simulink model "decoder8to256"  (R2020a)
settings: Solver=VariableStepAuto  StartTime=0.0  StopTime=10.0  RelTol=1e-3
(part 1 of 2)
settings Model: Creator=kishan  LastModifiedBy=kishan

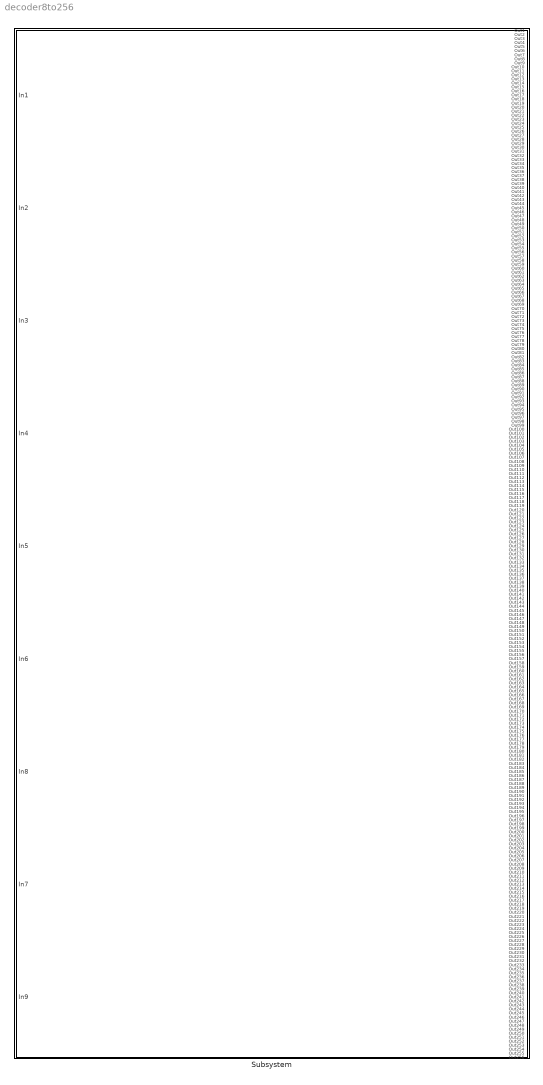
== system decoder8to256 ==
  Subsystem : Subsystem

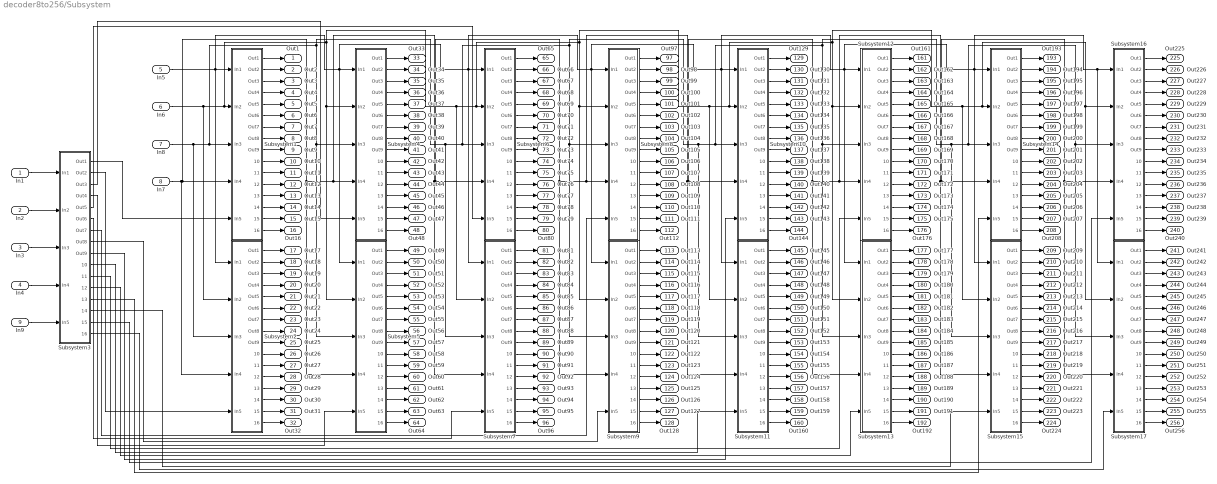
== system decoder8to256/Subsystem ==
  In1 : Inport
  In2 : Inport  Port=2
  In3 : Inport  Port=3
  In4 : Inport  Port=4
  In5 : Inport  Port=5
  In6 : Inport  Port=6
  In8 : Inport  Port=7
  In7 : Inport  Port=8
  In9 : Inport  Port=9
  Subsystem1 : Subsystem
  Subsystem10 : Subsystem
  Subsystem11 : Subsystem
  Subsystem12 : Subsystem
  Subsystem13 : Subsystem
  Subsystem14 : Subsystem
  Subsystem15 : Subsystem
  Subsystem16 : Subsystem
  Subsystem17 : Subsystem
  Subsystem2 : Subsystem
  Subsystem3 : Subsystem
  Subsystem4 : Subsystem
  Subsystem5 : Subsystem
  Subsystem6 : Subsystem
  Subsystem7 : Subsystem
  Subsystem8 : Subsystem
  Subsystem9 : Subsystem
  Out1 : Outport
  Out2 : Outport  Port=2
  Out3 : Outport  Port=3
  Out4 : Outport  Port=4
  Out5 : Outport  Port=5
  Out6 : Outport  Port=6
  Out7 : Outport  Port=7
  Out8 : Outport  Port=8
  Out9 : Outport  Port=9
  Out10 : Outport  Port=10
  Out11 : Outport  Port=11
  Out12 : Outport  Port=12
  Out13 : Outport  Port=13
  Out14 : Outport  Port=14
  Out15 : Outport  Port=15
  Out16 : Outport  Port=16
  Out17 : Outport  Port=17
  Out18 : Outport  Port=18
  Out19 : Outport  Port=19
  Out20 : Outport  Port=20
  Out21 : Outport  Port=21
  Out22 : Outport  Port=22
  Out23 : Outport  Port=23
  Out24 : Outport  Port=24
  Out25 : Outport  Port=25
  Out26 : Outport  Port=26
  Out27 : Outport  Port=27
  Out28 : Outport  Port=28
  Out29 : Outport  Port=29
  Out30 : Outport  Port=30
  Out31 : Outport  Port=31
  Out32 : Outport  Port=32
  Out33 : Outport  Port=33
  Out34 : Outport  Port=34
  Out35 : Outport  Port=35
  Out36 : Outport  Port=36
  Out37 : Outport  Port=37
  Out38 : Outport  Port=38
  Out39 : Outport  Port=39
  Out40 : Outport  Port=40
  Out41 : Outport  Port=41
  Out42 : Outport  Port=42
  Out43 : Outport  Port=43
  Out44 : Outport  Port=44
  Out45 : Outport  Port=45
  Out46 : Outport  Port=46
  Out47 : Outport  Port=47
  Out48 : Outport  Port=48
  Out49 : Outport  Port=49
  Out50 : Outport  Port=50
  Out51 : Outport  Port=51
  Out52 : Outport  Port=52
  Out53 : Outport  Port=53
  Out54 : Outport  Port=54
  Out55 : Outport  Port=55
  Out56 : Outport  Port=56
  Out57 : Outport  Port=57
  Out58 : Outport  Port=58
  Out59 : Outport  Port=59
  Out60 : Outport  Port=60
  Out61 : Outport  Port=61
  Out62 : Outport  Port=62
  Out63 : Outport  Port=63
  Out64 : Outport  Port=64
  Out65 : Outport  Port=65
  Out66 : Outport  Port=66
  Out67 : Outport  Port=67
  Out68 : Outport  Port=68
  Out69 : Outport  Port=69
  Out70 : Outport  Port=70
  Out71 : Outport  Port=71
  Out72 : Outport  Port=72
  Out73 : Outport  Port=73
  Out74 : Outport  Port=74
  Out75 : Outport  Port=75
  Out76 : Outport  Port=76
  Out77 : Outport  Port=77
  Out78 : Outport  Port=78
  Out79 : Outport  Port=79
  Out80 : Outport  Port=80
  Out81 : Outport  Port=81
  Out82 : Outport  Port=82
  Out83 : Outport  Port=83
  Out84 : Outport  Port=84
  Out85 : Outport  Port=85
  Out86 : Outport  Port=86
  Out87 : Outport  Port=87
  Out88 : Outport  Port=88
  Out89 : Outport  Port=89
  Out90 : Outport  Port=90
  Out91 : Outport  Port=91
  Out92 : Outport  Port=92
  Out93 : Outport  Port=93
  Out94 : Outport  Port=94
  Out95 : Outport  Port=95
  Out96 : Outport  Port=96
  Out97 : Outport  Port=97
  Out98 : Outport  Port=98
  Out99 : Outport  Port=99
  Out100 : Outport  Port=100
  Out101 : Outport  Port=101
  Out102 : Outport  Port=102
  Out103 : Outport  Port=103
  Out104 : Outport  Port=104
  Out105 : Outport  Port=105
  Out106 : Outport  Port=106
  Out107 : Outport  Port=107
  Out108 : Outport  Port=108
  Out109 : Outport  Port=109
  Out110 : Outport  Port=110
  Out111 : Outport  Port=111
  Out112 : Outport  Port=112
  Out113 : Outport  Port=113
  Out114 : Outport  Port=114
  Out115 : Outport  Port=115
  Out116 : Outport  Port=116
  Out117 : Outport  Port=117
  Out118 : Outport  Port=118
  Out119 : Outport  Port=119
  Out120 : Outport  Port=120
  Out121 : Outport  Port=121
  Out122 : Outport  Port=122
  Out123 : Outport  Port=123
  Out124 : Outport  Port=124
  Out125 : Outport  Port=125
  Out126 : Outport  Port=126
  Out127 : Outport  Port=127
  Out128 : Outport  Port=128
  Out129 : Outport  Port=129
  Out130 : Outport  Port=130
  Out131 : Outport  Port=131
  Out132 : Outport  Port=132
  Out133 : Outport  Port=133
  Out134 : Outport  Port=134
  Out135 : Outport  Port=135
  Out136 : Outport  Port=136
  Out137 : Outport  Port=137
  Out138 : Outport  Port=138
  Out139 : Outport  Port=139
  Out140 : Outport  Port=140
  Out141 : Outport  Port=141
  Out142 : Outport  Port=142
  Out143 : Outport  Port=143
  Out144 : Outport  Port=144
  Out145 : Outport  Port=145
  Out146 : Outport  Port=146
  Out147 : Outport  Port=147
  Out148 : Outport  Port=148
  Out149 : Outport  Port=149
  Out150 : Outport  Port=150
  Out151 : Outport  Port=151
  Out152 : Outport  Port=152
  Out153 : Outport  Port=153
  Out154 : Outport  Port=154
  Out155 : Outport  Port=155
  Out156 : Outport  Port=156
  Out157 : Outport  Port=157
  Out158 : Outport  Port=158
  Out159 : Outport  Port=159
  Out160 : Outport  Port=160
  Out161 : Outport  Port=161
  Out162 : Outport  Port=162
  Out163 : Outport  Port=163
  Out164 : Outport  Port=164
  Out165 : Outport  Port=165
  Out166 : Outport  Port=166
  Out167 : Outport  Port=167
  Out168 : Outport  Port=168
  Out169 : Outport  Port=169
  Out170 : Outport  Port=170
  Out171 : Outport  Port=171
  Out172 : Outport  Port=172
  Out173 : Outport  Port=173
  Out174 : Outport  Port=174
  Out175 : Outport  Port=175
  Out176 : Outport  Port=176
  Out177 : Outport  Port=177
  Out178 : Outport  Port=178
  Out179 : Outport  Port=179
  Out180 : Outport  Port=180
  Out181 : Outport  Port=181
  Out182 : Outport  Port=182
  Out183 : Outport  Port=183
  Out184 : Outport  Port=184
  Out185 : Outport  Port=185
  Out186 : Outport  Port=186
  Out187 : Outport  Port=187
  Out188 : Outport  Port=188
  Out189 : Outport  Port=189
  Out190 : Outport  Port=190
  Out191 : Outport  Port=191
  Out192 : Outport  Port=192
  Out193 : Outport  Port=193
  Out194 : Outport  Port=194
  Out195 : Outport  Port=195
  Out196 : Outport  Port=196
  Out197 : Outport  Port=197
  Out198 : Outport  Port=198
  Out199 : Outport  Port=199
  Out200 : Outport  Port=200
  Out201 : Outport  Port=201
  Out202 : Outport  Port=202
  Out203 : Outport  Port=203
  Out204 : Outport  Port=204
  Out205 : Outport  Port=205
  Out206 : Outport  Port=206
  Out207 : Outport  Port=207
  Out208 : Outport  Port=208
  Out209 : Outport  Port=209
  Out210 : Outport  Port=210
  Out211 : Outport  Port=211
  Out212 : Outport  Port=212
  Out213 : Outport  Port=213
  Out214 : Outport  Port=214
  Out215 : Outport  Port=215
  Out216 : Outport  Port=216
  Out217 : Outport  Port=217
  Out218 : Outport  Port=218
  Out219 : Outport  Port=219
  Out220 : Outport  Port=220
  Out221 : Outport  Port=221
  Out222 : Outport  Port=222
  Out223 : Outport  Port=223
  Out224 : Outport  Port=224
  Out225 : Outport  Port=225
  Out226 : Outport  Port=226
  Out227 : Outport  Port=227
  Out228 : Outport  Port=228
  Out229 : Outport  Port=229
  Out230 : Outport  Port=230
  Out231 : Outport  Port=231
  Out232 : Outport  Port=232
  Out233 : Outport  Port=233
  Out234 : Outport  Port=234
  Out235 : Outport  Port=235
  Out236 : Outport  Port=236
  Out237 : Outport  Port=237
  Out238 : Outport  Port=238
  Out239 : Outport  Port=239
  Out240 : Outport  Port=240
  Out241 : Outport  Port=241
  Out242 : Outport  Port=242
  Out243 : Outport  Port=243
  Out244 : Outport  Port=244
  Out245 : Outport  Port=245
  Out246 : Outport  Port=246
  Out247 : Outport  Port=247
  Out248 : Outport  Port=248
  Out249 : Outport  Port=249
  Out250 : Outport  Port=250
  Out251 : Outport  Port=251
  Out252 : Outport  Port=252
  Out253 : Outport  Port=253
  Out254 : Outport  Port=254
  Out255 : Outport  Port=255
  Out256 : Outport  Port=256
  wires:
  Subsystem17/5(Out5) -> Out245/1
  Subsystem15/13(Out13) -> Out221/1
  Subsystem5/12(Out12) -> Out60/1
  Subsystem6/8(Out8) -> Out72/1
  Subsystem10/7(Out7) -> Out135/1
  Subsystem13/13(Out13) -> Out189/1
  Subsystem14/10(Out10) -> Out202/1
  Subsystem11/5(Out5) -> Out149/1
  Subsystem10/5(Out5) -> Out133/1
  Subsystem7/14(Out14) -> Out94/1
  Subsystem7/2(Out2) -> Out82/1
  Subsystem12/7(Out7) -> Out167/1
  Subsystem7/10(Out10) -> Out90/1
  Subsystem8/12(Out12) -> Out108/1
  Subsystem12/1(Out1) -> Out161/1
  Subsystem17/4(Out4) -> Out244/1
  Subsystem7/15(Out15) -> Out95/1
  Subsystem10/13(Out13) -> Out141/1
  Subsystem3/12(Out12) -> Subsystem13/5(In5)
  Subsystem5/14(Out14) -> Out62/1
  Subsystem15/15(Out15) -> Out223/1
  Subsystem6/11(Out11) -> Out75/1
  Subsystem14/16(Out16) -> Out208/1
  Subsystem6/2(Out2) -> Out66/1
  Subsystem7/16(Out16) -> Out96/1
  Subsystem13/12(Out12) -> Out188/1
  Subsystem8/9(Out9) -> Out105/1
  Subsystem11/16(Out16) -> Out160/1
  Subsystem4/7(Out7) -> Out39/1
  Subsystem6/3(Out3) -> Out67/1
  In2/1 -> Subsystem3/2(In2)
  In4/1 -> Subsystem3/4(In4)
  Subsystem1/4(Out4) -> Out4/1
  Subsystem8/1(Out1) -> Out97/1
  Subsystem6/9(Out9) -> Out73/1
  Subsystem11/15(Out15) -> Out159/1
  Subsystem11/6(Out6) -> Out150/1
  Subsystem3/9(Out9) -> Subsystem10/5(In5)
  Subsystem17/10(Out10) -> Out250/1
  Subsystem9/4(Out4) -> Out116/1
  Subsystem9/8(Out8) -> Out120/1
  Subsystem11/7(Out7) -> Out151/1
  Subsystem9/6(Out6) -> Out118/1
  Subsystem4/4(Out4) -> Out36/1
  Subsystem16/1(Out1) -> Out225/1
  Subsystem9/14(Out14) -> Out126/1
  Subsystem7/4(Out4) -> Out84/1
  Subsystem9/16(Out16) -> Out128/1
  Subsystem1/14(Out14) -> Out14/1
  Subsystem12/14(Out14) -> Out174/1
  Subsystem6/12(Out12) -> Out76/1
  Subsystem16/11(Out11) -> Out235/1
  Subsystem15/12(Out12) -> Out220/1
  Subsystem8/7(Out7) -> Out103/1
  Subsystem13/6(Out6) -> Out182/1
  Subsystem5/4(Out4) -> Out52/1
  Subsystem14/8(Out8) -> Out200/1
  Subsystem14/1(Out1) -> Out193/1
  Subsystem11/3(Out3) -> Out147/1
  Subsystem16/16(Out16) -> Out240/1
  Subsystem4/6(Out6) -> Out38/1
  Subsystem5/6(Out6) -> Out54/1
  Subsystem15/16(Out16) -> Out224/1
  Subsystem2/14(Out14) -> Out30/1
  Subsystem3/7(Out7) -> Subsystem8/5(In5)
  Subsystem3/2(Out2) -> Subsystem2/5(In5)
  Subsystem13/2(Out2) -> Out178/1
  Subsystem7/7(Out7) -> Out87/1
  Subsystem1/3(Out3) -> Out3/1
  Subsystem4/3(Out3) -> Out35/1
  Subsystem11/2(Out2) -> Out146/1
  In5/1 -> Subsystem17/1(In1), Subsystem16/1(In1), Subsystem15/1(In1), Subsystem14/1(In1), Subsystem13/1(In1), Subsystem12/1(In1), Subsystem11/1(In1), Subsystem10/1(In1), Subsystem9/1(In1), Subsystem8/1(In1), Subsystem7/1(In1), Subsystem6/1(In1), Subsystem5/1(In1), Subsystem4/1(In1), Subsystem2/1(In1), Subsystem1/1(In1)
  Subsystem17/15(Out15) -> Out255/1
  Subsystem8/13(Out13) -> Out109/1
  Subsystem3/14(Out14) -> Subsystem15/5(In5)
  Subsystem3/10(Out10) -> Subsystem11/5(In5)
  Subsystem13/5(Out5) -> Out181/1
  Subsystem14/11(Out11) -> Out203/1
  Subsystem6/4(Out4) -> Out68/1
  Subsystem10/6(Out6) -> Out134/1
  Subsystem2/3(Out3) -> Out19/1
  Subsystem12/9(Out9) -> Out169/1
  Subsystem2/9(Out9) -> Out25/1
  Subsystem13/16(Out16) -> Out192/1
  Subsystem3/8(Out8) -> Subsystem9/5(In5)
  Subsystem15/8(Out8) -> Out216/1
  Subsystem14/4(Out4) -> Out196/1
  Subsystem5/8(Out8) -> Out56/1
  Subsystem9/12(Out12) -> Out124/1
  Subsystem16/7(Out7) -> Out231/1
  Subsystem9/1(Out1) -> Out113/1
  Subsystem16/3(Out3) -> Out227/1
  Subsystem13/15(Out15) -> Out191/1
  Subsystem17/2(Out2) -> Out242/1
  Subsystem1/6(Out6) -> Out6/1
  Subsystem2/4(Out4) -> Out20/1
  Subsystem16/8(Out8) -> Out232/1
  In3/1 -> Subsystem3/3(In3)
  Subsystem1/8(Out8) -> Out8/1
  Subsystem4/9(Out9) -> Out41/1
  Subsystem5/5(Out5) -> Out53/1
  Subsystem17/8(Out8) -> Out248/1
  Subsystem7/1(Out1) -> Out81/1
  Subsystem14/6(Out6) -> Out198/1
  Subsystem2/10(Out10) -> Out26/1
  Subsystem15/1(Out1) -> Out209/1
  Subsystem17/3(Out3) -> Out243/1
  Subsystem9/3(Out3) -> Out115/1
  Subsystem3/6(Out6) -> Subsystem7/5(In5)
  Subsystem7/13(Out13) -> Out93/1
  Subsystem17/12(Out12) -> Out252/1
  Subsystem9/2(Out2) -> Out114/1
  Subsystem6/16(Out16) -> Out80/1
  Subsystem11/13(Out13) -> Out157/1
  Subsystem10/1(Out1) -> Out129/1
  Subsystem7/9(Out9) -> Out89/1
  Subsystem15/6(Out6) -> Out214/1
  Subsystem17/11(Out11) -> Out251/1
  Subsystem12/16(Out16) -> Out176/1
  Subsystem4/12(Out12) -> Out44/1
  Subsystem2/5(Out5) -> Out21/1
  Subsystem8/16(Out16) -> Out112/1
  Subsystem16/4(Out4) -> Out228/1
  Subsystem6/10(Out10) -> Out74/1
  Subsystem5/16(Out16) -> Out64/1
  Subsystem5/11(Out11) -> Out59/1
  Subsystem1/12(Out12) -> Out12/1
  Subsystem11/12(Out12) -> Out156/1
  Subsystem1/7(Out7) -> Out7/1
  Subsystem14/13(Out13) -> Out205/1
  Subsystem2/15(Out15) -> Out31/1
  Subsystem10/10(Out10) -> Out138/1
  Subsystem13/4(Out4) -> Out180/1
  Subsystem11/10(Out10) -> Out154/1
  Subsystem11/1(Out1) -> Out145/1
  Subsystem3/16(Out16) -> Subsystem17/5(In5)
  Subsystem7/6(Out6) -> Out86/1
  Subsystem13/7(Out7) -> Out183/1
  Subsystem6/5(Out5) -> Out69/1
  Subsystem16/6(Out6) -> Out230/1
  Subsystem10/15(Out15) -> Out143/1
  Subsystem17/1(Out1) -> Out241/1
  Subsystem9/5(Out5) -> Out117/1
  Subsystem16/5(Out5) -> Out229/1
  Subsystem16/9(Out9) -> Out233/1
  Subsystem14/9(Out9) -> Out201/1
  Subsystem4/8(Out8) -> Out40/1
  Subsystem1/5(Out5) -> Out5/1
  Subsystem14/12(Out12) -> Out204/1
  Subsystem9/7(Out7) -> Out119/1
  Subsystem17/14(Out14) -> Out254/1
  Subsystem14/15(Out15) -> Out207/1
  Subsystem15/10(Out10) -> Out218/1
  Subsystem9/13(Out13) -> Out125/1
  Subsystem2/6(Out6) -> Out22/1
  Subsystem11/9(Out9) -> Out153/1
  Subsystem16/2(Out2) -> Out226/1
  Subsystem12/2(Out2) -> Out162/1
  Subsystem15/11(Out11) -> Out219/1
  Subsystem14/5(Out5) -> Out197/1
  Subsystem13/11(Out11) -> Out187/1
  In9/1 -> Subsystem3/5(In5)
  Subsystem16/12(Out12) -> Out236/1
  Subsystem1/1(Out1) -> Out1/1
  Subsystem12/13(Out13) -> Out173/1
  Subsystem9/9(Out9) -> Out121/1
  Subsystem17/9(Out9) -> Out249/1
  Subsystem12/10(Out10) -> Out170/1
  Subsystem15/3(Out3) -> Out211/1
  Subsystem3/13(Out13) -> Subsystem14/5(In5)
  Subsystem4/14(Out14) -> Out46/1
  In7/1 -> Subsystem17/4(In4), Subsystem16/4(In4), Subsystem14/4(In4), Subsystem15/4(In4), Subsystem12/4(In4), Subsystem13/4(In4), Subsystem10/4(In4), Subsystem11/4(In4), Subsystem8/4(In4), Subsystem9/4(In4), Subsystem6/4(In4), Subsystem7/4(In4), Subsystem4/4(In4), Subsystem5/4(In4), Subsystem1/4(In4), Subsystem2/4(In4)
  Subsystem15/9(Out9) -> Out217/1
  Subsystem10/3(Out3) -> Out131/1
  Subsystem1/11(Out11) -> Out11/1
  Subsystem6/14(Out14) -> Out78/1
  Subsystem5/2(Out2) -> Out50/1
  Subsystem10/16(Out16) -> Out144/1
  Subsystem5/9(Out9) -> Out57/1
  Subsystem1/10(Out10) -> Out10/1
  Subsystem14/7(Out7) -> Out199/1
  Subsystem8/5(Out5) -> Out101/1
  Subsystem16/10(Out10) -> Out234/1
  Subsystem15/4(Out4) -> Out212/1
  Subsystem17/6(Out6) -> Out246/1
  Subsystem12/11(Out11) -> Out171/1
  Subsystem12/6(Out6) -> Out166/1
  Subsystem9/11(Out11) -> Out123/1
  Subsystem1/13(Out13) -> Out13/1
  Subsystem5/3(Out3) -> Out51/1
  Subsystem8/14(Out14) -> Out110/1
  Subsystem4/5(Out5) -> Out37/1
  Subsystem17/16(Out16) -> Out256/1
  Subsystem10/9(Out9) -> Out137/1
  Subsystem17/7(Out7) -> Out247/1
  Subsystem13/8(Out8) -> Out184/1
  Subsystem4/2(Out2) -> Out34/1
  Subsystem3/4(Out4) -> Subsystem5/5(In5)
  Subsystem11/4(Out4) -> Out148/1
  Subsystem10/14(Out14) -> Out142/1
  Subsystem4/11(Out11) -> Out43/1
  Subsystem8/15(Out15) -> Out111/1
  Subsystem2/7(Out7) -> Out23/1
  Subsystem9/15(Out15) -> Out127/1
  Subsystem3/1(Out1) -> Subsystem1/5(In5)
  Subsystem5/13(Out13) -> Out61/1
  Subsystem6/13(Out13) -> Out77/1
  Subsystem16/14(Out14) -> Out238/1
  Subsystem13/10(Out10) -> Out186/1
  In8/1 -> Subsystem1/3(In3), Subsystem5/3(In3), Subsystem4/3(In3), Subsystem6/3(In3), Subsystem9/3(In3), Subsystem8/3(In3), Subsystem10/3(In3), Subsystem13/3(In3), Subsystem12/3(In3), Subsystem14/3(In3), Subsystem17/3(In3), Subsystem16/3(In3), Subsystem15/3(In3), Subsystem11/3(In3), Subsystem7/3(In3), Subsystem2/3(In3)
  Subsystem1/15(Out15) -> Out15/1
  Subsystem12/15(Out15) -> Out175/1
  Subsystem8/10(Out10) -> Out106/1
  Subsystem7/8(Out8) -> Out88/1
  Subsystem2/1(Out1) -> Out17/1
  Subsystem10/2(Out2) -> Out130/1
  Subsystem11/11(Out11) -> Out155/1
  Subsystem12/5(Out5) -> Out165/1
  Subsystem9/10(Out10) -> Out122/1
  Subsystem1/2(Out2) -> Out2/1
  Subsystem6/6(Out6) -> Out70/1
  Subsystem4/16(Out16) -> Out48/1
  Subsystem2/8(Out8) -> Out24/1
  Subsystem2/12(Out12) -> Out28/1
  Subsystem6/15(Out15) -> Out79/1
  Subsystem8/3(Out3) -> Out99/1
  Subsystem17/13(Out13) -> Out253/1
  Subsystem15/14(Out14) -> Out222/1
  Subsystem7/5(Out5) -> Out85/1
  Subsystem8/2(Out2) -> Out98/1
  Subsystem14/2(Out2) -> Out194/1
  Subsystem13/1(Out1) -> Out177/1
  Subsystem15/5(Out5) -> Out213/1
  Subsystem11/14(Out14) -> Out158/1
  Subsystem10/8(Out8) -> Out136/1
  Subsystem13/14(Out14) -> Out190/1
  In6/1 -> Subsystem5/2(In2), Subsystem4/2(In2), Subsystem9/2(In2), Subsystem8/2(In2), Subsystem13/2(In2), Subsystem12/2(In2), Subsystem17/2(In2), Subsystem16/2(In2), Subsystem14/2(In2), Subsystem15/2(In2), Subsystem10/2(In2), Subsystem11/2(In2), Subsystem6/2(In2), Subsystem7/2(In2), Subsystem1/2(In2), Subsystem2/2(In2)
  Subsystem11/8(Out8) -> Out152/1
  Subsystem8/6(Out6) -> Out102/1
  Subsystem8/4(Out4) -> Out100/1
  Subsystem15/7(Out7) -> Out215/1
  Subsystem4/15(Out15) -> Out47/1
  Subsystem12/12(Out12) -> Out172/1
  Subsystem15/2(Out2) -> Out210/1
  Subsystem16/13(Out13) -> Out237/1
  Subsystem6/1(Out1) -> Out65/1
  Subsystem16/15(Out15) -> Out239/1
  Subsystem12/3(Out3) -> Out163/1
  Subsystem5/10(Out10) -> Out58/1
  In1/1 -> Subsystem3/1(In1)
  Subsystem13/3(Out3) -> Out179/1
  Subsystem5/7(Out7) -> Out55/1
  Subsystem3/3(Out3) -> Subsystem4/5(In5)
  Subsystem4/13(Out13) -> Out45/1
  Subsystem2/2(Out2) -> Out18/1
  Subsystem2/16(Out16) -> Out32/1
  Subsystem4/10(Out10) -> Out42/1
  Subsystem7/12(Out12) -> Out92/1
  Subsystem1/16(Out16) -> Out16/1
  Subsystem2/11(Out11) -> Out27/1
  Subsystem10/11(Out11) -> Out139/1
  Subsystem12/4(Out4) -> Out164/1
  Subsystem14/3(Out3) -> Out195/1
  Subsystem5/1(Out1) -> Out49/1
  Subsystem8/11(Out11) -> Out107/1
  Subsystem10/12(Out12) -> Out140/1
  Subsystem2/13(Out13) -> Out29/1
  Subsystem12/8(Out8) -> Out168/1
  Subsystem1/9(Out9) -> Out9/1
  Subsystem10/4(Out4) -> Out132/1
  Subsystem13/9(Out9) -> Out185/1
  Subsystem3/15(Out15) -> Subsystem16/5(In5)
  Subsystem7/3(Out3) -> Out83/1
  Subsystem6/7(Out7) -> Out71/1
  Subsystem7/11(Out11) -> Out91/1
  Subsystem5/15(Out15) -> Out63/1
  Subsystem3/11(Out11) -> Subsystem12/5(In5)
  Subsystem14/14(Out14) -> Out206/1
  Subsystem4/1(Out1) -> Out33/1
  Subsystem3/5(Out5) -> Subsystem6/5(In5)
  Subsystem8/8(Out8) -> Out104/1

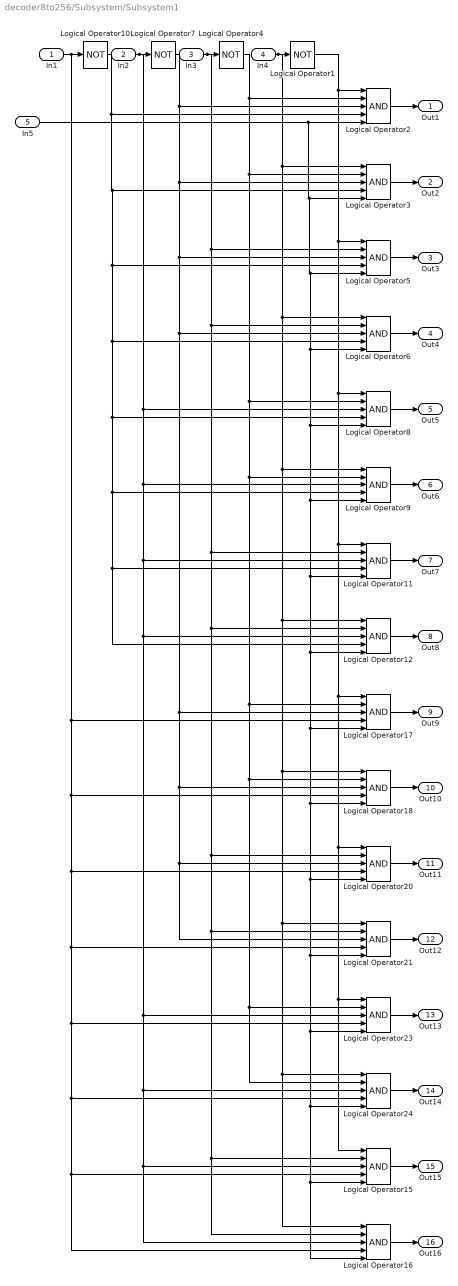
== system decoder8to256/Subsystem/Subsystem1 ==
  In1 : Inport
  In2 : Inport  Port=2
  In3 : Inport  Port=3
  In4 : Inport  Port=4
  In5 : Inport  Port=5
  Logical Operator{1,4,7,10} (4 alike) : Logic  Operator=NOT  AllPortsSameDT=off  OutDataTypeStr=boolean
  Logical Operator{2..3,5..6,8..9,11..12,15..18,20..21,23..24} (16 alike) : Logic  Inputs=5  AllPortsSameDT=off  OutDataTypeStr=boolean
  Out1 : Outport
  Out2 : Outport  Port=2
  Out3 : Outport  Port=3
  Out4 : Outport  Port=4
  Out5 : Outport  Port=5
  Out6 : Outport  Port=6
  Out7 : Outport  Port=7
  Out8 : Outport  Port=8
  Out9 : Outport  Port=9
  Out10 : Outport  Port=10
  Out11 : Outport  Port=11
  Out12 : Outport  Port=12
  Out13 : Outport  Port=13
  Out14 : Outport  Port=14
  Out15 : Outport  Port=15
  Out16 : Outport  Port=16
  wires:
  Logical Operator11/1 -> Out7/1
  Logical Operator12/1 -> Out8/1
  Logical Operator18/1 -> Out10/1
  In2/1 -> Logical Operator16/3, Logical Operator15/3, Logical Operator24/3, Logical Operator23/3, Logical Operator12/3, Logical Operator11/3, Logical Operator9/3, Logical Operator8/3, Logical Operator7/1
  In3/1 -> Logical Operator11/2, Logical Operator15/2, Logical Operator16/2, Logical Operator21/2, Logical Operator20/2, Logical Operator12/2, Logical Operator6/2, Logical Operator5/2, Logical Operator4/1
  Logical Operator24/1 -> Out14/1
  In4/1 -> Logical Operator16/1, Logical Operator24/1, Logical Operator21/1, Logical Operator18/1, Logical Operator12/1, Logical Operator9/1, Logical Operator6/1, Logical Operator3/1, Logical Operator1/1
  Logical Operator10/1 -> Logical Operator12/4, Logical Operator11/4, Logical Operator9/4, Logical Operator8/4, Logical Operator6/4, Logical Operator5/4, Logical Operator3/4, Logical Operator2/4
  Logical Operator9/1 -> Out6/1
  In5/1 -> Logical Operator16/5, Logical Operator15/5, Logical Operator24/5, Logical Operator23/5, Logical Operator21/5, Logical Operator20/5, Logical Operator18/5, Logical Operator17/5, Logical Operator12/5, Logical Operator11/5, Logical Operator9/5, Logical Operator8/5, Logical Operator6/5, Logical Operator5/5, Logical Operator3/5, Logical Operator2/5
  Logical Operator5/1 -> Out3/1
  Logical Operator1/1 -> Logical Operator15/1, Logical Operator23/1, Logical Operator20/1, Logical Operator17/1, Logical Operator11/1, Logical Operator8/1, Logical Operator5/1, Logical Operator2/1
  Logical Operator2/1 -> Out1/1
  Logical Operator21/1 -> Out12/1
  Logical Operator8/1 -> Out5/1
  Logical Operator7/1 -> Logical Operator21/3, Logical Operator20/3, Logical Operator18/3, Logical Operator17/3, Logical Operator6/3, Logical Operator5/3, Logical Operator3/3, Logical Operator2/3
  Logical Operator16/1 -> Out16/1
  Logical Operator15/1 -> Out15/1
  In1/1 -> Logical Operator17/4, Logical Operator18/4, Logical Operator20/4, Logical Operator21/4, Logical Operator23/4, Logical Operator24/4, Logical Operator15/4, Logical Operator16/4, Logical Operator10/1
  Logical Operator3/1 -> Out2/1
  Logical Operator20/1 -> Out11/1
  Logical Operator6/1 -> Out4/1
  Logical Operator23/1 -> Out13/1
  Logical Operator4/1 -> Logical Operator24/2, Logical Operator23/2, Logical Operator18/2, Logical Operator17/2, Logical Operator9/2, Logical Operator8/2, Logical Operator3/2, Logical Operator2/2
  Logical Operator17/1 -> Out9/1

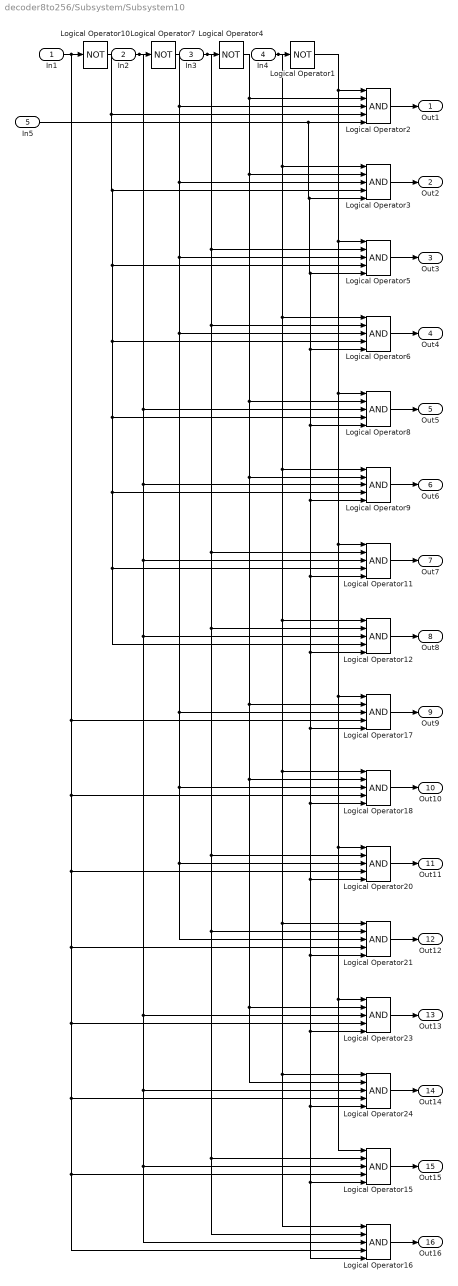
== system decoder8to256/Subsystem/Subsystem10 ==
  In1 : Inport
  In2 : Inport  Port=2
  In3 : Inport  Port=3
  In4 : Inport  Port=4
  In5 : Inport  Port=5
  Logical Operator{1,4,7,10} (4 alike) : Logic  Operator=NOT  AllPortsSameDT=off  OutDataTypeStr=boolean
  Logical Operator{2..3,5..6,8..9,11..12,15..18,20..21,23..24} (16 alike) : Logic  Inputs=5  AllPortsSameDT=off  OutDataTypeStr=boolean
  Out1 : Outport
  Out2 : Outport  Port=2
  Out3 : Outport  Port=3
  Out4 : Outport  Port=4
  Out5 : Outport  Port=5
  Out6 : Outport  Port=6
  Out7 : Outport  Port=7
  Out8 : Outport  Port=8
  Out9 : Outport  Port=9
  Out10 : Outport  Port=10
  Out11 : Outport  Port=11
  Out12 : Outport  Port=12
  Out13 : Outport  Port=13
  Out14 : Outport  Port=14
  Out15 : Outport  Port=15
  Out16 : Outport  Port=16
  wires:
  Logical Operator11/1 -> Out7/1
  Logical Operator12/1 -> Out8/1
  Logical Operator18/1 -> Out10/1
  In2/1 -> Logical Operator16/3, Logical Operator15/3, Logical Operator24/3, Logical Operator23/3, Logical Operator12/3, Logical Operator11/3, Logical Operator9/3, Logical Operator8/3, Logical Operator7/1
  In3/1 -> Logical Operator11/2, Logical Operator15/2, Logical Operator16/2, Logical Operator21/2, Logical Operator20/2, Logical Operator12/2, Logical Operator6/2, Logical Operator5/2, Logical Operator4/1
  Logical Operator24/1 -> Out14/1
  In4/1 -> Logical Operator16/1, Logical Operator24/1, Logical Operator21/1, Logical Operator18/1, Logical Operator12/1, Logical Operator9/1, Logical Operator6/1, Logical Operator3/1, Logical Operator1/1
  Logical Operator10/1 -> Logical Operator12/4, Logical Operator11/4, Logical Operator9/4, Logical Operator8/4, Logical Operator6/4, Logical Operator5/4, Logical Operator3/4, Logical Operator2/4
  Logical Operator9/1 -> Out6/1
  In5/1 -> Logical Operator16/5, Logical Operator15/5, Logical Operator24/5, Logical Operator23/5, Logical Operator21/5, Logical Operator20/5, Logical Operator18/5, Logical Operator17/5, Logical Operator12/5, Logical Operator11/5, Logical Operator9/5, Logical Operator8/5, Logical Operator6/5, Logical Operator5/5, Logical Operator3/5, Logical Operator2/5
  Logical Operator5/1 -> Out3/1
  Logical Operator1/1 -> Logical Operator15/1, Logical Operator23/1, Logical Operator20/1, Logical Operator17/1, Logical Operator11/1, Logical Operator8/1, Logical Operator5/1, Logical Operator2/1
  Logical Operator2/1 -> Out1/1
  Logical Operator21/1 -> Out12/1
  Logical Operator8/1 -> Out5/1
  Logical Operator7/1 -> Logical Operator21/3, Logical Operator20/3, Logical Operator18/3, Logical Operator17/3, Logical Operator6/3, Logical Operator5/3, Logical Operator3/3, Logical Operator2/3
  Logical Operator16/1 -> Out16/1
  Logical Operator15/1 -> Out15/1
  In1/1 -> Logical Operator17/4, Logical Operator18/4, Logical Operator20/4, Logical Operator21/4, Logical Operator23/4, Logical Operator24/4, Logical Operator15/4, Logical Operator16/4, Logical Operator10/1
  Logical Operator3/1 -> Out2/1
  Logical Operator20/1 -> Out11/1
  Logical Operator6/1 -> Out4/1
  Logical Operator23/1 -> Out13/1
  Logical Operator4/1 -> Logical Operator24/2, Logical Operator23/2, Logical Operator18/2, Logical Operator17/2, Logical Operator9/2, Logical Operator8/2, Logical Operator3/2, Logical Operator2/2
  Logical Operator17/1 -> Out9/1

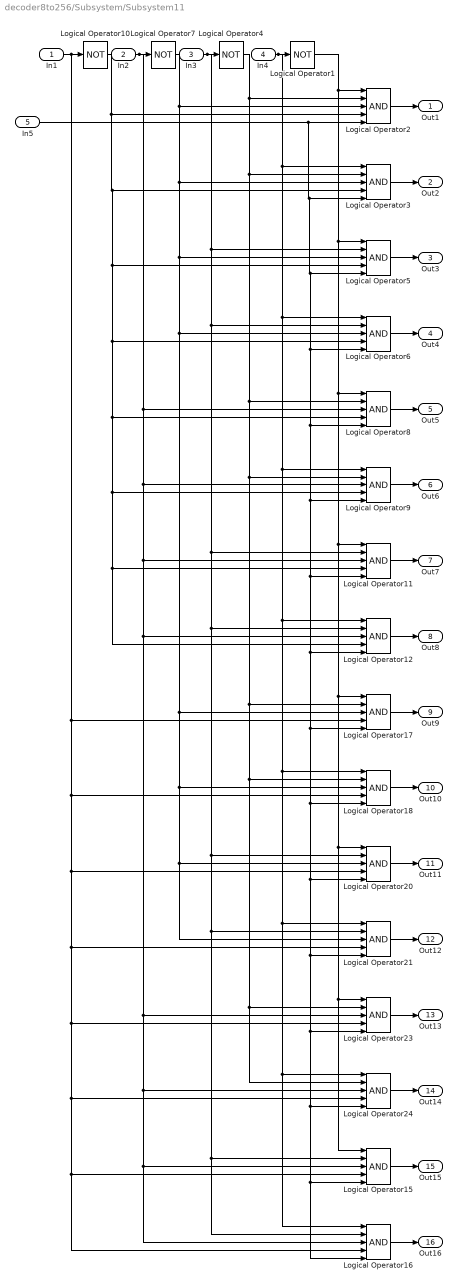
== system decoder8to256/Subsystem/Subsystem11 ==
  In1 : Inport
  In2 : Inport  Port=2
  In3 : Inport  Port=3
  In4 : Inport  Port=4
  In5 : Inport  Port=5
  Logical Operator{1,4,7,10} (4 alike) : Logic  Operator=NOT  AllPortsSameDT=off  OutDataTypeStr=boolean
  Logical Operator{2..3,5..6,8..9,11..12,15..18,20..21,23..24} (16 alike) : Logic  Inputs=5  AllPortsSameDT=off  OutDataTypeStr=boolean
  Out1 : Outport
  Out2 : Outport  Port=2
  Out3 : Outport  Port=3
  Out4 : Outport  Port=4
  Out5 : Outport  Port=5
  Out6 : Outport  Port=6
  Out7 : Outport  Port=7
  Out8 : Outport  Port=8
  Out9 : Outport  Port=9
  Out10 : Outport  Port=10
  Out11 : Outport  Port=11
  Out12 : Outport  Port=12
  Out13 : Outport  Port=13
  Out14 : Outport  Port=14
  Out15 : Outport  Port=15
  Out16 : Outport  Port=16
  wires:
  Logical Operator11/1 -> Out7/1
  Logical Operator12/1 -> Out8/1
  Logical Operator18/1 -> Out10/1
  In2/1 -> Logical Operator16/3, Logical Operator15/3, Logical Operator24/3, Logical Operator23/3, Logical Operator12/3, Logical Operator11/3, Logical Operator9/3, Logical Operator8/3, Logical Operator7/1
  In3/1 -> Logical Operator11/2, Logical Operator15/2, Logical Operator16/2, Logical Operator21/2, Logical Operator20/2, Logical Operator12/2, Logical Operator6/2, Logical Operator5/2, Logical Operator4/1
  Logical Operator24/1 -> Out14/1
  In4/1 -> Logical Operator16/1, Logical Operator24/1, Logical Operator21/1, Logical Operator18/1, Logical Operator12/1, Logical Operator9/1, Logical Operator6/1, Logical Operator3/1, Logical Operator1/1
  Logical Operator10/1 -> Logical Operator12/4, Logical Operator11/4, Logical Operator9/4, Logical Operator8/4, Logical Operator6/4, Logical Operator5/4, Logical Operator3/4, Logical Operator2/4
  Logical Operator9/1 -> Out6/1
  In5/1 -> Logical Operator16/5, Logical Operator15/5, Logical Operator24/5, Logical Operator23/5, Logical Operator21/5, Logical Operator20/5, Logical Operator18/5, Logical Operator17/5, Logical Operator12/5, Logical Operator11/5, Logical Operator9/5, Logical Operator8/5, Logical Operator6/5, Logical Operator5/5, Logical Operator3/5, Logical Operator2/5
  Logical Operator5/1 -> Out3/1
  Logical Operator1/1 -> Logical Operator15/1, Logical Operator23/1, Logical Operator20/1, Logical Operator17/1, Logical Operator11/1, Logical Operator8/1, Logical Operator5/1, Logical Operator2/1
  Logical Operator2/1 -> Out1/1
  Logical Operator21/1 -> Out12/1
  Logical Operator8/1 -> Out5/1
  Logical Operator7/1 -> Logical Operator21/3, Logical Operator20/3, Logical Operator18/3, Logical Operator17/3, Logical Operator6/3, Logical Operator5/3, Logical Operator3/3, Logical Operator2/3
  Logical Operator16/1 -> Out16/1
  Logical Operator15/1 -> Out15/1
  In1/1 -> Logical Operator17/4, Logical Operator18/4, Logical Operator20/4, Logical Operator21/4, Logical Operator23/4, Logical Operator24/4, Logical Operator15/4, Logical Operator16/4, Logical Operator10/1
  Logical Operator3/1 -> Out2/1
  Logical Operator20/1 -> Out11/1
  Logical Operator6/1 -> Out4/1
  Logical Operator23/1 -> Out13/1
  Logical Operator4/1 -> Logical Operator24/2, Logical Operator23/2, Logical Operator18/2, Logical Operator17/2, Logical Operator9/2, Logical Operator8/2, Logical Operator3/2, Logical Operator2/2
  Logical Operator17/1 -> Out9/1

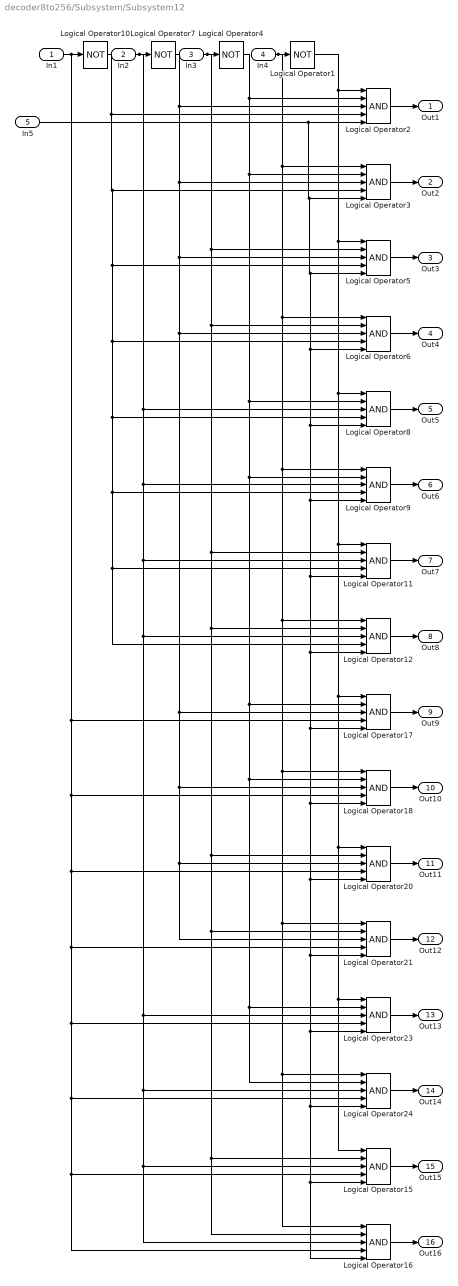
== system decoder8to256/Subsystem/Subsystem12 ==
  In1 : Inport
  In2 : Inport  Port=2
  In3 : Inport  Port=3
  In4 : Inport  Port=4
  In5 : Inport  Port=5
  Logical Operator{1,4,7,10} (4 alike) : Logic  Operator=NOT  AllPortsSameDT=off  OutDataTypeStr=boolean
  Logical Operator{2..3,5..6,8..9,11..12,15..18,20..21,23..24} (16 alike) : Logic  Inputs=5  AllPortsSameDT=off  OutDataTypeStr=boolean
  Out1 : Outport
  Out2 : Outport  Port=2
  Out3 : Outport  Port=3
  Out4 : Outport  Port=4
  Out5 : Outport  Port=5
  Out6 : Outport  Port=6
  Out7 : Outport  Port=7
  Out8 : Outport  Port=8
  Out9 : Outport  Port=9
  Out10 : Outport  Port=10
  Out11 : Outport  Port=11
  Out12 : Outport  Port=12
  Out13 : Outport  Port=13
  Out14 : Outport  Port=14
  Out15 : Outport  Port=15
  Out16 : Outport  Port=16
  wires:
  Logical Operator11/1 -> Out7/1
  Logical Operator12/1 -> Out8/1
  Logical Operator18/1 -> Out10/1
  In2/1 -> Logical Operator16/3, Logical Operator15/3, Logical Operator24/3, Logical Operator23/3, Logical Operator12/3, Logical Operator11/3, Logical Operator9/3, Logical Operator8/3, Logical Operator7/1
  In3/1 -> Logical Operator11/2, Logical Operator15/2, Logical Operator16/2, Logical Operator21/2, Logical Operator20/2, Logical Operator12/2, Logical Operator6/2, Logical Operator5/2, Logical Operator4/1
  Logical Operator24/1 -> Out14/1
  In4/1 -> Logical Operator16/1, Logical Operator24/1, Logical Operator21/1, Logical Operator18/1, Logical Operator12/1, Logical Operator9/1, Logical Operator6/1, Logical Operator3/1, Logical Operator1/1
  Logical Operator10/1 -> Logical Operator12/4, Logical Operator11/4, Logical Operator9/4, Logical Operator8/4, Logical Operator6/4, Logical Operator5/4, Logical Operator3/4, Logical Operator2/4
  Logical Operator9/1 -> Out6/1
  In5/1 -> Logical Operator16/5, Logical Operator15/5, Logical Operator24/5, Logical Operator23/5, Logical Operator21/5, Logical Operator20/5, Logical Operator18/5, Logical Operator17/5, Logical Operator12/5, Logical Operator11/5, Logical Operator9/5, Logical Operator8/5, Logical Operator6/5, Logical Operator5/5, Logical Operator3/5, Logical Operator2/5
  Logical Operator5/1 -> Out3/1
  Logical Operator1/1 -> Logical Operator15/1, Logical Operator23/1, Logical Operator20/1, Logical Operator17/1, Logical Operator11/1, Logical Operator8/1, Logical Operator5/1, Logical Operator2/1
  Logical Operator2/1 -> Out1/1
  Logical Operator21/1 -> Out12/1
  Logical Operator8/1 -> Out5/1
  Logical Operator7/1 -> Logical Operator21/3, Logical Operator20/3, Logical Operator18/3, Logical Operator17/3, Logical Operator6/3, Logical Operator5/3, Logical Operator3/3, Logical Operator2/3
  Logical Operator16/1 -> Out16/1
  Logical Operator15/1 -> Out15/1
  In1/1 -> Logical Operator17/4, Logical Operator18/4, Logical Operator20/4, Logical Operator21/4, Logical Operator23/4, Logical Operator24/4, Logical Operator15/4, Logical Operator16/4, Logical Operator10/1
  Logical Operator3/1 -> Out2/1
  Logical Operator20/1 -> Out11/1
  Logical Operator6/1 -> Out4/1
  Logical Operator23/1 -> Out13/1
  Logical Operator4/1 -> Logical Operator24/2, Logical Operator23/2, Logical Operator18/2, Logical Operator17/2, Logical Operator9/2, Logical Operator8/2, Logical Operator3/2, Logical Operator2/2
  Logical Operator17/1 -> Out9/1

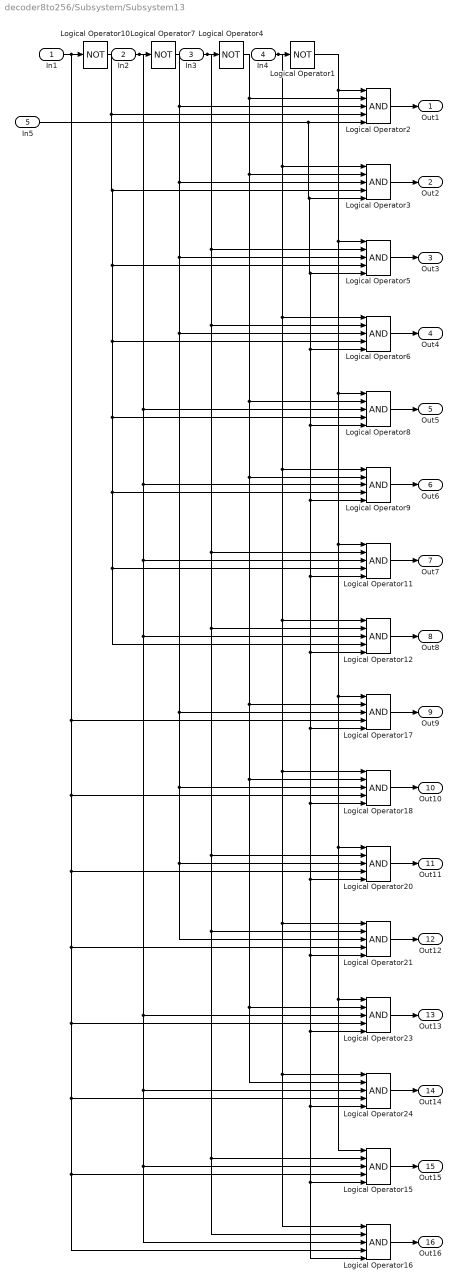
== system decoder8to256/Subsystem/Subsystem13 ==
  In1 : Inport
  In2 : Inport  Port=2
  In3 : Inport  Port=3
  In4 : Inport  Port=4
  In5 : Inport  Port=5
  Logical Operator{1,4,7,10} (4 alike) : Logic  Operator=NOT  AllPortsSameDT=off  OutDataTypeStr=boolean
  Logical Operator{2..3,5..6,8..9,11..12,15..18,20..21,23..24} (16 alike) : Logic  Inputs=5  AllPortsSameDT=off  OutDataTypeStr=boolean
  Out1 : Outport
  Out2 : Outport  Port=2
  Out3 : Outport  Port=3
  Out4 : Outport  Port=4
  Out5 : Outport  Port=5
  Out6 : Outport  Port=6
  Out7 : Outport  Port=7
  Out8 : Outport  Port=8
  Out9 : Outport  Port=9
  Out10 : Outport  Port=10
  Out11 : Outport  Port=11
  Out12 : Outport  Port=12
  Out13 : Outport  Port=13
  Out14 : Outport  Port=14
  Out15 : Outport  Port=15
  Out16 : Outport  Port=16
  wires:
  Logical Operator11/1 -> Out7/1
  Logical Operator12/1 -> Out8/1
  Logical Operator18/1 -> Out10/1
  In2/1 -> Logical Operator16/3, Logical Operator15/3, Logical Operator24/3, Logical Operator23/3, Logical Operator12/3, Logical Operator11/3, Logical Operator9/3, Logical Operator8/3, Logical Operator7/1
  In3/1 -> Logical Operator11/2, Logical Operator15/2, Logical Operator16/2, Logical Operator21/2, Logical Operator20/2, Logical Operator12/2, Logical Operator6/2, Logical Operator5/2, Logical Operator4/1
  Logical Operator24/1 -> Out14/1
  In4/1 -> Logical Operator16/1, Logical Operator24/1, Logical Operator21/1, Logical Operator18/1, Logical Operator12/1, Logical Operator9/1, Logical Operator6/1, Logical Operator3/1, Logical Operator1/1
  Logical Operator10/1 -> Logical Operator12/4, Logical Operator11/4, Logical Operator9/4, Logical Operator8/4, Logical Operator6/4, Logical Operator5/4, Logical Operator3/4, Logical Operator2/4
  Logical Operator9/1 -> Out6/1
  In5/1 -> Logical Operator16/5, Logical Operator15/5, Logical Operator24/5, Logical Operator23/5, Logical Operator21/5, Logical Operator20/5, Logical Operator18/5, Logical Operator17/5, Logical Operator12/5, Logical Operator11/5, Logical Operator9/5, Logical Operator8/5, Logical Operator6/5, Logical Operator5/5, Logical Operator3/5, Logical Operator2/5
  Logical Operator5/1 -> Out3/1
  Logical Operator1/1 -> Logical Operator15/1, Logical Operator23/1, Logical Operator20/1, Logical Operator17/1, Logical Operator11/1, Logical Operator8/1, Logical Operator5/1, Logical Operator2/1
  Logical Operator2/1 -> Out1/1
  Logical Operator21/1 -> Out12/1
  Logical Operator8/1 -> Out5/1
  Logical Operator7/1 -> Logical Operator21/3, Logical Operator20/3, Logical Operator18/3, Logical Operator17/3, Logical Operator6/3, Logical Operator5/3, Logical Operator3/3, Logical Operator2/3
  Logical Operator16/1 -> Out16/1
  Logical Operator15/1 -> Out15/1
  In1/1 -> Logical Operator17/4, Logical Operator18/4, Logical Operator20/4, Logical Operator21/4, Logical Operator23/4, Logical Operator24/4, Logical Operator15/4, Logical Operator16/4, Logical Operator10/1
  Logical Operator3/1 -> Out2/1
  Logical Operator20/1 -> Out11/1
  Logical Operator6/1 -> Out4/1
  Logical Operator23/1 -> Out13/1
  Logical Operator4/1 -> Logical Operator24/2, Logical Operator23/2, Logical Operator18/2, Logical Operator17/2, Logical Operator9/2, Logical Operator8/2, Logical Operator3/2, Logical Operator2/2
  Logical Operator17/1 -> Out9/1

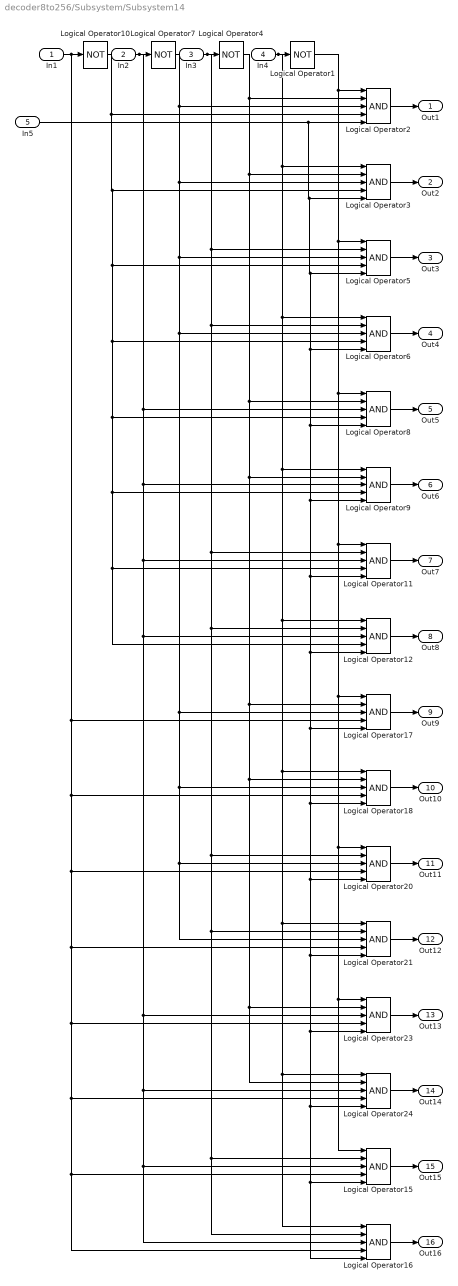
== system decoder8to256/Subsystem/Subsystem14 ==
  In1 : Inport
  In2 : Inport  Port=2
  In3 : Inport  Port=3
  In4 : Inport  Port=4
  In5 : Inport  Port=5
  Logical Operator{1,4,7,10} (4 alike) : Logic  Operator=NOT  AllPortsSameDT=off  OutDataTypeStr=boolean
  Logical Operator{2..3,5..6,8..9,11..12,15..18,20..21,23..24} (16 alike) : Logic  Inputs=5  AllPortsSameDT=off  OutDataTypeStr=boolean
  Out1 : Outport
  Out2 : Outport  Port=2
  Out3 : Outport  Port=3
  Out4 : Outport  Port=4
  Out5 : Outport  Port=5
  Out6 : Outport  Port=6
  Out7 : Outport  Port=7
  Out8 : Outport  Port=8
  Out9 : Outport  Port=9
  Out10 : Outport  Port=10
  Out11 : Outport  Port=11
  Out12 : Outport  Port=12
  Out13 : Outport  Port=13
  Out14 : Outport  Port=14
  Out15 : Outport  Port=15
  Out16 : Outport  Port=16
  wires:
  Logical Operator11/1 -> Out7/1
  Logical Operator12/1 -> Out8/1
  Logical Operator18/1 -> Out10/1
  In2/1 -> Logical Operator16/3, Logical Operator15/3, Logical Operator24/3, Logical Operator23/3, Logical Operator12/3, Logical Operator11/3, Logical Operator9/3, Logical Operator8/3, Logical Operator7/1
  In3/1 -> Logical Operator11/2, Logical Operator15/2, Logical Operator16/2, Logical Operator21/2, Logical Operator20/2, Logical Operator12/2, Logical Operator6/2, Logical Operator5/2, Logical Operator4/1
  Logical Operator24/1 -> Out14/1
  In4/1 -> Logical Operator16/1, Logical Operator24/1, Logical Operator21/1, Logical Operator18/1, Logical Operator12/1, Logical Operator9/1, Logical Operator6/1, Logical Operator3/1, Logical Operator1/1
  Logical Operator10/1 -> Logical Operator12/4, Logical Operator11/4, Logical Operator9/4, Logical Operator8/4, Logical Operator6/4, Logical Operator5/4, Logical Operator3/4, Logical Operator2/4
  Logical Operator9/1 -> Out6/1
  In5/1 -> Logical Operator16/5, Logical Operator15/5, Logical Operator24/5, Logical Operator23/5, Logical Operator21/5, Logical Operator20/5, Logical Operator18/5, Logical Operator17/5, Logical Operator12/5, Logical Operator11/5, Logical Operator9/5, Logical Operator8/5, Logical Operator6/5, Logical Operator5/5, Logical Operator3/5, Logical Operator2/5
  Logical Operator5/1 -> Out3/1
  Logical Operator1/1 -> Logical Operator15/1, Logical Operator23/1, Logical Operator20/1, Logical Operator17/1, Logical Operator11/1, Logical Operator8/1, Logical Operator5/1, Logical Operator2/1
  Logical Operator2/1 -> Out1/1
  Logical Operator21/1 -> Out12/1
  Logical Operator8/1 -> Out5/1
  Logical Operator7/1 -> Logical Operator21/3, Logical Operator20/3, Logical Operator18/3, Logical Operator17/3, Logical Operator6/3, Logical Operator5/3, Logical Operator3/3, Logical Operator2/3
  Logical Operator16/1 -> Out16/1
  Logical Operator15/1 -> Out15/1
  In1/1 -> Logical Operator17/4, Logical Operator18/4, Logical Operator20/4, Logical Operator21/4, Logical Operator23/4, Logical Operator24/4, Logical Operator15/4, Logical Operator16/4, Logical Operator10/1
  Logical Operator3/1 -> Out2/1
  Logical Operator20/1 -> Out11/1
  Logical Operator6/1 -> Out4/1
  Logical Operator23/1 -> Out13/1
  Logical Operator4/1 -> Logical Operator24/2, Logical Operator23/2, Logical Operator18/2, Logical Operator17/2, Logical Operator9/2, Logical Operator8/2, Logical Operator3/2, Logical Operator2/2
  Logical Operator17/1 -> Out9/1

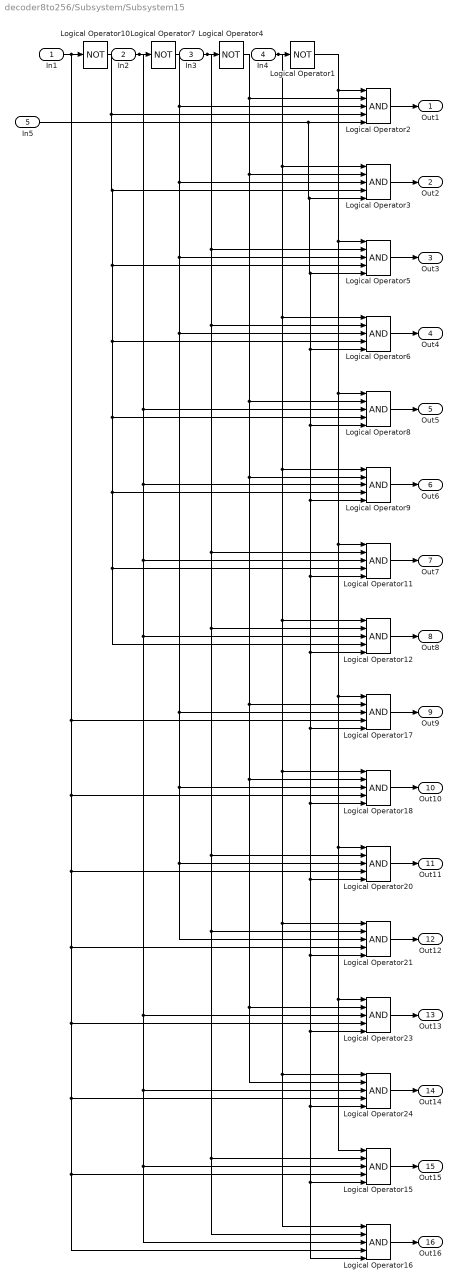
== system decoder8to256/Subsystem/Subsystem15 ==
  In1 : Inport
  In2 : Inport  Port=2
  In3 : Inport  Port=3
  In4 : Inport  Port=4
  In5 : Inport  Port=5
  Logical Operator{1,4,7,10} (4 alike) : Logic  Operator=NOT  AllPortsSameDT=off  OutDataTypeStr=boolean
  Logical Operator{2..3,5..6,8..9,11..12,15..18,20..21,23..24} (16 alike) : Logic  Inputs=5  AllPortsSameDT=off  OutDataTypeStr=boolean
  Out1 : Outport
  Out2 : Outport  Port=2
  Out3 : Outport  Port=3
  Out4 : Outport  Port=4
  Out5 : Outport  Port=5
  Out6 : Outport  Port=6
  Out7 : Outport  Port=7
  Out8 : Outport  Port=8
  Out9 : Outport  Port=9
  Out10 : Outport  Port=10
  Out11 : Outport  Port=11
  Out12 : Outport  Port=12
  Out13 : Outport  Port=13
  Out14 : Outport  Port=14
  Out15 : Outport  Port=15
  Out16 : Outport  Port=16
  wires:
  Logical Operator11/1 -> Out7/1
  Logical Operator12/1 -> Out8/1
  Logical Operator18/1 -> Out10/1
  In2/1 -> Logical Operator16/3, Logical Operator15/3, Logical Operator24/3, Logical Operator23/3, Logical Operator12/3, Logical Operator11/3, Logical Operator9/3, Logical Operator8/3, Logical Operator7/1
  In3/1 -> Logical Operator11/2, Logical Operator15/2, Logical Operator16/2, Logical Operator21/2, Logical Operator20/2, Logical Operator12/2, Logical Operator6/2, Logical Operator5/2, Logical Operator4/1
  Logical Operator24/1 -> Out14/1
  In4/1 -> Logical Operator16/1, Logical Operator24/1, Logical Operator21/1, Logical Operator18/1, Logical Operator12/1, Logical Operator9/1, Logical Operator6/1, Logical Operator3/1, Logical Operator1/1
  Logical Operator10/1 -> Logical Operator12/4, Logical Operator11/4, Logical Operator9/4, Logical Operator8/4, Logical Operator6/4, Logical Operator5/4, Logical Operator3/4, Logical Operator2/4
  Logical Operator9/1 -> Out6/1
  In5/1 -> Logical Operator16/5, Logical Operator15/5, Logical Operator24/5, Logical Operator23/5, Logical Operator21/5, Logical Operator20/5, Logical Operator18/5, Logical Operator17/5, Logical Operator12/5, Logical Operator11/5, Logical Operator9/5, Logical Operator8/5, Logical Operator6/5, Logical Operator5/5, Logical Operator3/5, Logical Operator2/5
  Logical Operator5/1 -> Out3/1
  Logical Operator1/1 -> Logical Operator15/1, Logical Operator23/1, Logical Operator20/1, Logical Operator17/1, Logical Operator11/1, Logical Operator8/1, Logical Operator5/1, Logical Operator2/1
  Logical Operator2/1 -> Out1/1
  Logical Operator21/1 -> Out12/1
  Logical Operator8/1 -> Out5/1
  Logical Operator7/1 -> Logical Operator21/3, Logical Operator20/3, Logical Operator18/3, Logical Operator17/3, Logical Operator6/3, Logical Operator5/3, Logical Operator3/3, Logical Operator2/3
  Logical Operator16/1 -> Out16/1
  Logical Operator15/1 -> Out15/1
  In1/1 -> Logical Operator17/4, Logical Operator18/4, Logical Operator20/4, Logical Operator21/4, Logical Operator23/4, Logical Operator24/4, Logical Operator15/4, Logical Operator16/4, Logical Operator10/1
  Logical Operator3/1 -> Out2/1
  Logical Operator20/1 -> Out11/1
  Logical Operator6/1 -> Out4/1
  Logical Operator23/1 -> Out13/1
  Logical Operator4/1 -> Logical Operator24/2, Logical Operator23/2, Logical Operator18/2, Logical Operator17/2, Logical Operator9/2, Logical Operator8/2, Logical Operator3/2, Logical Operator2/2
  Logical Operator17/1 -> Out9/1

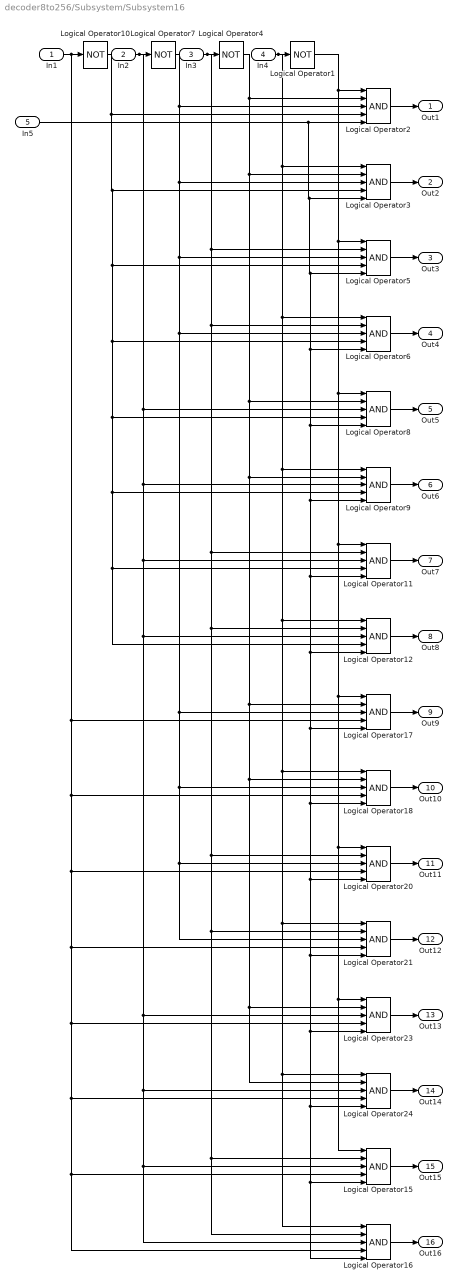
== system decoder8to256/Subsystem/Subsystem16 ==
  In1 : Inport
  In2 : Inport  Port=2
  In3 : Inport  Port=3
  In4 : Inport  Port=4
  In5 : Inport  Port=5
  Logical Operator{1,4,7,10} (4 alike) : Logic  Operator=NOT  AllPortsSameDT=off  OutDataTypeStr=boolean
  Logical Operator{2..3,5..6,8..9,11..12,15..18,20..21,23..24} (16 alike) : Logic  Inputs=5  AllPortsSameDT=off  OutDataTypeStr=boolean
  Out1 : Outport
  Out2 : Outport  Port=2
  Out3 : Outport  Port=3
  Out4 : Outport  Port=4
  Out5 : Outport  Port=5
  Out6 : Outport  Port=6
  Out7 : Outport  Port=7
  Out8 : Outport  Port=8
  Out9 : Outport  Port=9
  Out10 : Outport  Port=10
  Out11 : Outport  Port=11
  Out12 : Outport  Port=12
  Out13 : Outport  Port=13
  Out14 : Outport  Port=14
  Out15 : Outport  Port=15
  Out16 : Outport  Port=16
  wires:
  Logical Operator11/1 -> Out7/1
  Logical Operator12/1 -> Out8/1
  Logical Operator18/1 -> Out10/1
  In2/1 -> Logical Operator16/3, Logical Operator15/3, Logical Operator24/3, Logical Operator23/3, Logical Operator12/3, Logical Operator11/3, Logical Operator9/3, Logical Operator8/3, Logical Operator7/1
  In3/1 -> Logical Operator11/2, Logical Operator15/2, Logical Operator16/2, Logical Operator21/2, Logical Operator20/2, Logical Operator12/2, Logical Operator6/2, Logical Operator5/2, Logical Operator4/1
  Logical Operator24/1 -> Out14/1
  In4/1 -> Logical Operator16/1, Logical Operator24/1, Logical Operator21/1, Logical Operator18/1, Logical Operator12/1, Logical Operator9/1, Logical Operator6/1, Logical Operator3/1, Logical Operator1/1
  Logical Operator10/1 -> Logical Operator12/4, Logical Operator11/4, Logical Operator9/4, Logical Operator8/4, Logical Operator6/4, Logical Operator5/4, Logical Operator3/4, Logical Operator2/4
  Logical Operator9/1 -> Out6/1
  In5/1 -> Logical Operator16/5, Logical Operator15/5, Logical Operator24/5, Logical Operator23/5, Logical Operator21/5, Logical Operator20/5, Logical Operator18/5, Logical Operator17/5, Logical Operator12/5, Logical Operator11/5, Logical Operator9/5, Logical Operator8/5, Logical Operator6/5, Logical Operator5/5, Logical Operator3/5, Logical Operator2/5
  Logical Operator5/1 -> Out3/1
  Logical Operator1/1 -> Logical Operator15/1, Logical Operator23/1, Logical Operator20/1, Logical Operator17/1, Logical Operator11/1, Logical Operator8/1, Logical Operator5/1, Logical Operator2/1
  Logical Operator2/1 -> Out1/1
  Logical Operator21/1 -> Out12/1
  Logical Operator8/1 -> Out5/1
  Logical Operator7/1 -> Logical Operator21/3, Logical Operator20/3, Logical Operator18/3, Logical Operator17/3, Logical Operator6/3, Logical Operator5/3, Logical Operator3/3, Logical Operator2/3
  Logical Operator16/1 -> Out16/1
  Logical Operator15/1 -> Out15/1
  In1/1 -> Logical Operator17/4, Logical Operator18/4, Logical Operator20/4, Logical Operator21/4, Logical Operator23/4, Logical Operator24/4, Logical Operator15/4, Logical Operator16/4, Logical Operator10/1
  Logical Operator3/1 -> Out2/1
  Logical Operator20/1 -> Out11/1
  Logical Operator6/1 -> Out4/1
  Logical Operator23/1 -> Out13/1
  Logical Operator4/1 -> Logical Operator24/2, Logical Operator23/2, Logical Operator18/2, Logical Operator17/2, Logical Operator9/2, Logical Operator8/2, Logical Operator3/2, Logical Operator2/2
  Logical Operator17/1 -> Out9/1

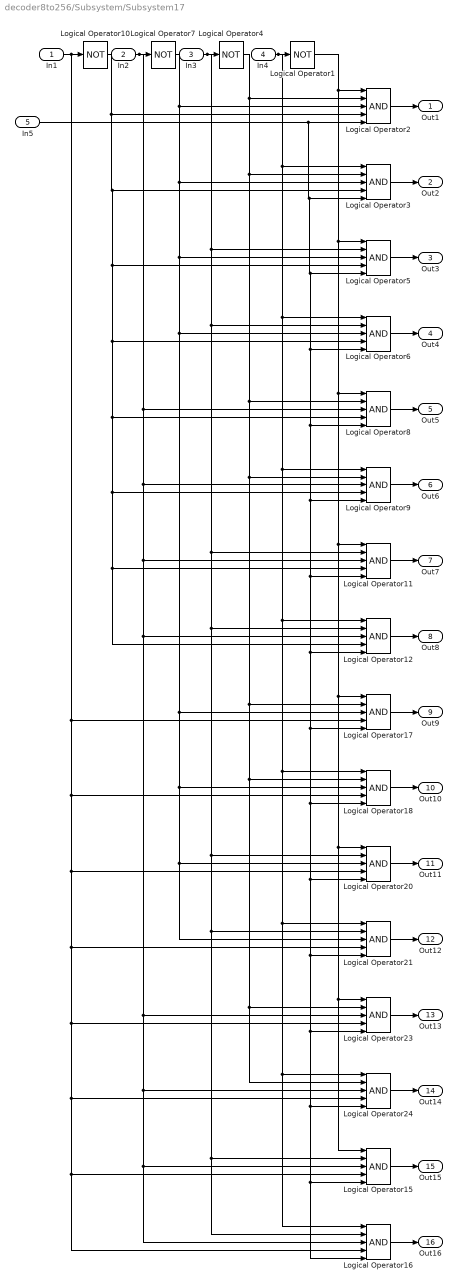
== system decoder8to256/Subsystem/Subsystem17 ==
  In1 : Inport
  In2 : Inport  Port=2
  In3 : Inport  Port=3
  In4 : Inport  Port=4
  In5 : Inport  Port=5
  Logical Operator{1,4,7,10} (4 alike) : Logic  Operator=NOT  AllPortsSameDT=off  OutDataTypeStr=boolean
  Logical Operator{2..3,5..6,8..9,11..12,15..18,20..21,23..24} (16 alike) : Logic  Inputs=5  AllPortsSameDT=off  OutDataTypeStr=boolean
  Out1 : Outport
  Out2 : Outport  Port=2
  Out3 : Outport  Port=3
  Out4 : Outport  Port=4
  Out5 : Outport  Port=5
  Out6 : Outport  Port=6
  Out7 : Outport  Port=7
  Out8 : Outport  Port=8
  Out9 : Outport  Port=9
  Out10 : Outport  Port=10
  Out11 : Outport  Port=11
  Out12 : Outport  Port=12
  Out13 : Outport  Port=13
  Out14 : Outport  Port=14
  Out15 : Outport  Port=15
  Out16 : Outport  Port=16
  wires:
  Logical Operator11/1 -> Out7/1
  Logical Operator12/1 -> Out8/1
  Logical Operator18/1 -> Out10/1
  In2/1 -> Logical Operator16/3, Logical Operator15/3, Logical Operator24/3, Logical Operator23/3, Logical Operator12/3, Logical Operator11/3, Logical Operator9/3, Logical Operator8/3, Logical Operator7/1
  In3/1 -> Logical Operator11/2, Logical Operator15/2, Logical Operator16/2, Logical Operator21/2, Logical Operator20/2, Logical Operator12/2, Logical Operator6/2, Logical Operator5/2, Logical Operator4/1
  Logical Operator24/1 -> Out14/1
  In4/1 -> Logical Operator16/1, Logical Operator24/1, Logical Operator21/1, Logical Operator18/1, Logical Operator12/1, Logical Operator9/1, Logical Operator6/1, Logical Operator3/1, Logical Operator1/1
  Logical Operator10/1 -> Logical Operator12/4, Logical Operator11/4, Logical Operator9/4, Logical Operator8/4, Logical Operator6/4, Logical Operator5/4, Logical Operator3/4, Logical Operator2/4
  Logical Operator9/1 -> Out6/1
  In5/1 -> Logical Operator16/5, Logical Operator15/5, Logical Operator24/5, Logical Operator23/5, Logical Operator21/5, Logical Operator20/5, Logical Operator18/5, Logical Operator17/5, Logical Operator12/5, Logical Operator11/5, Logical Operator9/5, Logical Operator8/5, Logical Operator6/5, Logical Operator5/5, Logical Operator3/5, Logical Operator2/5
  Logical Operator5/1 -> Out3/1
  Logical Operator1/1 -> Logical Operator15/1, Logical Operator23/1, Logical Operator20/1, Logical Operator17/1, Logical Operator11/1, Logical Operator8/1, Logical Operator5/1, Logical Operator2/1
  Logical Operator2/1 -> Out1/1
  Logical Operator21/1 -> Out12/1
  Logical Operator8/1 -> Out5/1
  Logical Operator7/1 -> Logical Operator21/3, Logical Operator20/3, Logical Operator18/3, Logical Operator17/3, Logical Operator6/3, Logical Operator5/3, Logical Operator3/3, Logical Operator2/3
  Logical Operator16/1 -> Out16/1
  Logical Operator15/1 -> Out15/1
  In1/1 -> Logical Operator17/4, Logical Operator18/4, Logical Operator20/4, Logical Operator21/4, Logical Operator23/4, Logical Operator24/4, Logical Operator15/4, Logical Operator16/4, Logical Operator10/1
  Logical Operator3/1 -> Out2/1
  Logical Operator20/1 -> Out11/1
  Logical Operator6/1 -> Out4/1
  Logical Operator23/1 -> Out13/1
  Logical Operator4/1 -> Logical Operator24/2, Logical Operator23/2, Logical Operator18/2, Logical Operator17/2, Logical Operator9/2, Logical Operator8/2, Logical Operator3/2, Logical Operator2/2
  Logical Operator17/1 -> Out9/1
